simulink model "first_model"  (R2016a)
settings: Solver=VariableStepAuto  StartTime=0.0  StopTime=5  RelTol=1e-3
libraries: powerlib x17, powerlib_meascontrol x4
settings Model: Creator=St  LastModifiedBy=Mac

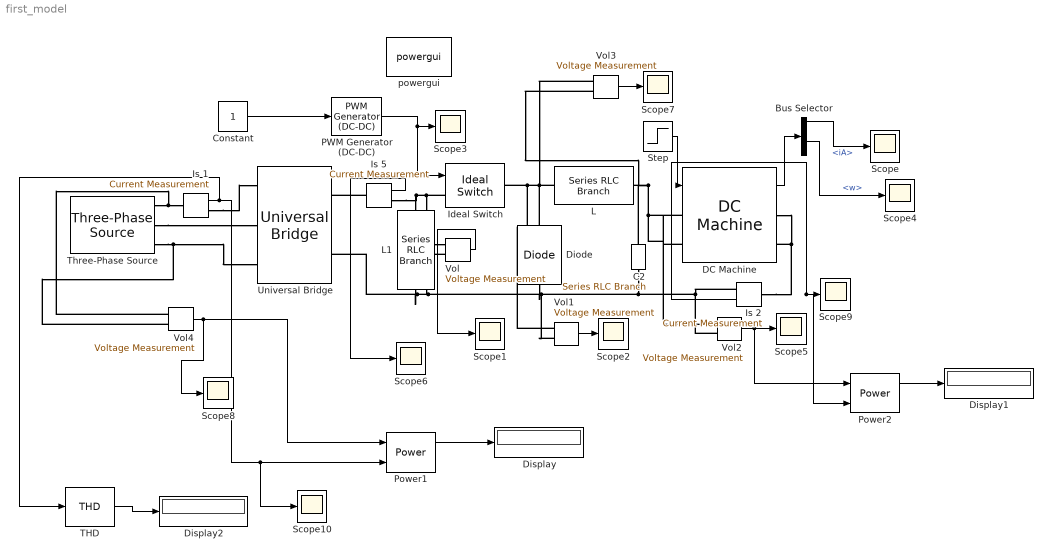
== system first_model ==
  Bus Selector : BusSelector  OutputSignals=iA,iF,w,Te
  C2 : powerlib/Elements/Series RLC Branch  LConnTagsString=__new0  RConnTagsString=__new0  BranchType=C  Resistance=1  Inductance=1e-3  SetiL0=off  InitialCurrent=0  Capacitance=1e-5  Setx0=off  InitialVoltage=0  Measurements=None
  Constant : Constant
  DC Machine : powerlib/Machines/DC Machine  PresetModel=No  MechanicalLoad=Torque TL  FieldType=Wound  ShowDetailedParameters=on  MeasurementBus=on  RLa=[ 28 0.0133]  RLf="[ 8260  6.4]"  Laf=1.8  MachineConstant=Torque constant (N.m/A)  Ke=1.8  Kt=1.8  J=1  Bm=0  Tf=0  w0=1  Ifinit=1  TsPowergui=0  TsBlock=-1
  Diode : powerlib/Power Electronics/Diode  Ron=1e-8  Lon=0  Vf=0  IC=0  UseSnubber=off  Rs=500  Cs=250e-9  Measurements=off
  Display : Display
  Display1 : Display
  Display2 : Display
  Ideal Switch : powerlib/Power Electronics/Ideal Switch  Ron=0.001  Lon=0  IC=0  Rs=1e5  Cs=inf  Measurements=off
  Is 1 : powerlib/Measurements/Current Measurement  PhasorSimulation=off  OutputType=Complex  PSBequivalent=0
  Is 2 : powerlib/Measurements/Current Measurement  PhasorSimulation=off  OutputType=Complex  PSBequivalent=0
  Is 5 : powerlib/Measurements/Current Measurement  PhasorSimulation=off  OutputType=Complex  PSBequivalent=0
  L : powerlib/Elements/Series RLC Branch  LConnTagsString=__new0  RConnTagsString=__new0  BranchType=L  Resistance=1  Inductance=0.01  SetiL0=off  InitialCurrent=0  Capacitance=1e-6  Setx0=off  InitialVoltage=0  Measurements=None
  L1 : powerlib/Elements/Series RLC Branch  LConnTagsString=__new0  RConnTagsString=__new0  BranchType=C  Resistance=1  Inductance=0.01  SetiL0=off  InitialCurrent=0  Capacitance=680e-6  Setx0=off  InitialVoltage=0  Measurements=None
  PWM Generator (DC-DC) : powerlib_meascontrol/Pulse & Signal Generators/PWM Generator (DC-DC)  Fsw=4000  Ts=0
  Power1 : powerlib_meascontrol/Measurements/Power  Freq=50  Vinit=[1, 0]  Iinit=[1, 0]  Ts=0.1
  Power2 : powerlib_meascontrol/Measurements/Power  Freq=50  Vinit=[1, 0]  Iinit=[1, 0]  Ts=0.1
  Scope{,1..10} (11 alike) : Scope
  Step : Step  Time=10  After=0  SampleTime=0
  THD : powerlib_meascontrol/Measurements/THD  Freq=60  Ts=0
  Three-Phase Source : powerlib/Electrical Sources/Three-Phase Source  InternalConnection=Yg  VoltagePhases=off  Voltage=220/sqrt(2)  PhaseAngle=0  Voltage_phases=[25e3 25e3 25e3]/sqrt(3)  PhaseAngles_phases=[0 -120 +120]  Frequency=50  NonIdealSource=off  SpecifyImpedance=off  Resistance=0.8929  Inductance=16.58e-3  ShortCircuitLevel=100e6  BaseVoltage=25e3  XRratio=7  BusType=swing  Pref=10e3  Qref=0  Prefabc=[10e3, 10e3, 10e3]  Qrefabc=[0, 0, 0]  Qmin=-inf  Qmax=inf
  Universal Bridge : powerlib/Power Electronics/Universal Bridge  Arms=3  SnubberResistance=1e5  SnubberCapacitance=inf  Device=Diodes  Ron=1e-3  Lon=0  ForwardVoltages="[  0  0  ]"  ForwardVoltage=0  GTOparameters=[ 10e-6 , 20e-6 ]  IGBTparameters=[ 1e-6 , 2e-6 ]  Measurements=None  Measurements_2=None  converterType=Rectifier
  Vol{,1..4} (5 alike) : powerlib/Measurements/Voltage Measurement  PhasorSimulation=off  OutputType=Complex  PSBequivalent=0
  powergui : powerlib/powergui  Priority=1  SimulationMode=Continuous  SolverType=Tustin/Backward Euler (TBE)  SampleTime=50e-7  frequency=60  SPID=off  DisableSnubberDevices=off  DisableRonSwitches=off  DisableVfSwitches=off  SwTol=0  DisplayEquations=off  Interpol=off  ExternalGateDelay=off  methode=off  Ts=10  FunctionMessages=off  echomessages=off  HookPort=off  EnableUseOfTLC=off  x0status=blocks  frequencyindice=50  Pbase=100e6  ErrMax=1e-4  Iterations=50  UnitsV=kV  UnitsW=MW  buscounter=0  RestoreLinks=warning  ResistiveCurrentMeasurement=off  Frange=[0:2:500]  Ylog=off  Xlog=on  ShowGrid=off  save=off  variable=ZData  structure=0  ZoomFFT=off  StartTime=0.0  cycles=1  DisplayStyle=1  fundamental=60  FreqAxis=off  MaxFrequency=1000  frequencyindicesteady=1  RmsSteady=1  display=off
  wires:
  PWM Generator (DC-DC)/1 -> Scope3/1, Ideal Switch/1
  Constant/1 -> PWM Generator (DC-DC)/1
  DC Machine/1 -> Bus Selector/1
  Bus Selector/1 -> Scope/1  "<iA>"
  Vol/1 -> Scope1/1
  Vol1/1 -> Scope2/1
  Step/1 -> DC Machine/1
  Bus Selector/3 -> Scope4/1  "<w>"
  Vol2/1 -> Power2/1, Scope5/1
  Is 5/1 -> Scope6/1
  Vol3/1 -> Scope7/1
  Vol4/1 -> Scope8/1, Power1/1
  Power1/1 -> Display/1
  Is 1/1 -> THD/1, Scope10/1, Power1/2
  Is 2/1 -> Power2/2, Scope9/1
  Power2/1 -> Display1/1
  THD/1 -> Display2/1
  connections:
  Three-Phase Source/RConn2 -- Universal Bridge/LConn2
  Three-Phase Source/RConn3 -- Vol4/LConn2 -- Universal Bridge/LConn3
  L/LConn1 -- Vol3/LConn1 -- Diode/RConn1 -- Ideal Switch/RConn1 -- Vol1/LConn1
  Vol2/LConn2 -- Is 2/RConn1 -- C2/RConn1 -- Diode/LConn1 -- Universal Bridge/RConn2 -- L1/RConn1 -- Vol/LConn2 -- Vol1/LConn2
  DC Machine/LConn1 -- Vol2/LConn1 -- DC Machine/LConn2 -- C2/LConn1 -- Vol3/LConn2 -- L/RConn1
  Ideal Switch/LConn1 -- Is 5/RConn1 -- L1/LConn1 -- Vol/LConn1
  Is 5/LConn1 -- Universal Bridge/RConn1
  Is 1/RConn1 -- Universal Bridge/LConn1
  Three-Phase Source/RConn1 -- Vol4/LConn1 -- Is 1/LConn1
  DC Machine/RConn1 -- Is 2/LConn1 -- DC Machine/RConn2
